simulink model "power_FCV_powertrain_modified"  (R2021b)
settings: Solver=ode23tb  StartTime=0.0  StopTime=1175  RelTol=1e-3  EnableMultiTasking=on
PreLoadFcn:
  | Ts=60e-6;
InitFcn:
  | Pbatt = 25e3;
  | Vbatt = 288;
values from neighbouring files (symbols this model uses):
  Cr = 0.013    [datavehicule.m]    (also in workspace.mat)
  Cx = 0.25    [datavehicule.m]    (also in workspace.mat = 0.65)
  efficency_FC = 0.53    [init.m]    (also in main.m; workspace.mat)
  epsilon = 10^-6    (= 1e-06)    [init.m]    (also in workspace.mat)
  g = 9.81    [datavehicule.m]    (also in init.m; workspace.mat)
  gr = 17/64    (= 0.265625)    [datavehicule.m]    (also in workspace.mat)
  M = 1400    [datavehicule.m]    (also in workspace.mat = 2000)
  p = 0    [datavehicule.m]    (also in workspace.mat)
  Pbatt_2 = 25000    [workspace.mat]
  ro = 1.23    [datavehicule.m]    (also in workspace.mat)
  Sf = 1.6+0.00056*(M-765)    [ForceTrac.m]    (also in workspace.mat = 3.93)
  V = [t, velocity]    [init.m]
undefined symbols (not defined in the file or in its folder): DiscIntNeverNeededParam, Ion, Lithium
libraries: simulink x9, sdl_lib x8, spsCurrentMeasurementLib x6, fl_lib x6, nesl_utility x6, spsSeriesRLCBranchLib x4, AC6DriveInternalModels x3, simulink_extras x2, spsBatteryLib x1, DC6DriveInternalModels x1, spsDiodeLib x1, spsFuelCellStackLib x1
(part 2 of 2)

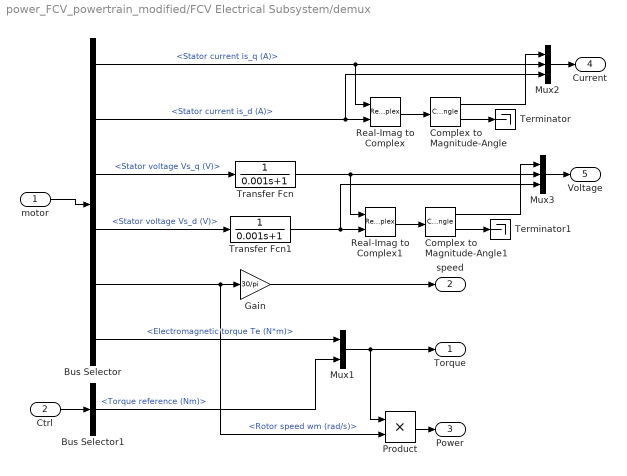
== system power_FCV_powertrain_modified/FCV Electrical Subsystem/demux ==
  motor : Inport
  Ctrl : Inport  Port=2
  Bus Selector : BusSelector  OutputSignals=Stator current is_q (A),Stator current is_d (A),Stator voltage Vs_q (V),Stator voltage Vs_d (V),Rotor speed wm (rad/s),Electromagnetic torque Te (N*m)
  Bus Selector1 : BusSelector  OutputSignals=Torque reference (Nm)
  Complex to Magnitude-Angle : ComplexToMagnitudeAngle
  Complex to Magnitude-Angle1 : ComplexToMagnitudeAngle
  Gain : Gain  Gain=30/pi  SaturateOnIntegerOverflow=on  OutDataTypeStr=Inherit: Same as input  ParamDataTypeStr=Inherit: Same as input
  Mux1 : Mux  Inputs=2
  Mux2 : Mux  Inputs=3
  Mux3 : Mux  Inputs=3
  Product : Product  RndMeth=Zero
  Real-Imag to Complex : RealImagToComplex
  Real-Imag to Complex1 : RealImagToComplex
  Terminator : Terminator
  Terminator1 : Terminator
  Transfer Fcn : TransferFcn  Denominator=[0.001 1]
  Transfer Fcn1 : TransferFcn  Denominator=[0.001 1]
  Torque : Outport
  speed : Outport  Port=2
  Power : Outport  Port=3
  Current : Outport  Port=4
  Voltage : Outport  Port=5
  wires:
  Bus Selector/5 -> Gain/1, Product/2  "<Rotor speed wm (rad/s)>"
  Ctrl/1 -> Bus Selector1/1
  Gain/1 -> speed/1
  Mux1/1 -> Torque/1, Product/1
  motor/1 -> Bus Selector/1
  Mux2/1 -> Current/1
  Product/1 -> Power/1
  Bus Selector/2 -> Real-Imag to Complex/2, Mux2/3  "<Stator current is_d (A)>"
  Bus Selector/1 -> Real-Imag to Complex/1, Mux2/2  "<Stator current is_q (A)>"
  Real-Imag to Complex/1 -> Complex to Magnitude-Angle/1
  Complex to Magnitude-Angle/2 -> Terminator/1
  Complex to Magnitude-Angle/1 -> Mux2/1
  Mux3/1 -> Voltage/1
  Bus Selector/4 -> Transfer Fcn1/1  "<Stator voltage Vs_d (V)>"
  Bus Selector/3 -> Transfer Fcn/1  "<Stator voltage Vs_q (V)>"
  Real-Imag to Complex1/1 -> Complex to Magnitude-Angle1/1
  Complex to Magnitude-Angle1/2 -> Terminator1/1
  Complex to Magnitude-Angle1/1 -> Mux3/1
  Transfer Fcn/1 -> Mux3/2, Real-Imag to Complex1/1
  Transfer Fcn1/1 -> Mux3/3, Real-Imag to Complex1/2
  Bus Selector/6 -> Mux1/1  "<Electromagnetic torque Te (N*m)>"
  Bus Selector1/1 -> Mux1/2  "<Torque reference (Nm)>"

== system power_FCV_powertrain_modified/Energy Management Subsystem/Power Management System/Battery Available Power ==
  P FC : Inport
  P* FC : Inport  Port=2
  Battery recharge : Inport  Port=3
  Power limit : Inport  Port=4
  Add2 : Sum  Inputs=-+
  Compare To Zero : simulink/Logic and Bit Operations/Compare To Zero  relop=~=  OutDataTypeStr=boolean
  Gain : Gain  Gain=-1
  Rate Limiter : RateLimiter  RisingSlewLimit=Pbatt  FallingSlewLimit=-Pbatt  SampleTimeMode=inherited
  Saturation Dynamic : simulink/Discontinuities/Saturation Dynamic  OutMin=[]  OutMax=[]  OutDataTypeStr=Inherit: Same as second input  OutDataType=sfix(16)  OutScaling=2^-10  DoSatur=off
  Switch1 : Switch  Criteria=u2 ~= 0
  Switch2 : Switch  Criteria=u2 ~= 0
  Battery power : Outport
  wires:
  Battery recharge/1 -> Switch1/1, Compare To Zero/1
  Compare To Zero/1 -> Switch1/2, Switch2/2
  P FC/1 -> Add2/1
  Saturation Dynamic/1 -> Battery power/1
  P* FC/1 -> Add2/2
  Add2/1 -> Switch1/3, Switch2/3  "P batt"
  Power limit/1 -> Gain/1, Saturation Dynamic/1
  Gain/1 -> Saturation Dynamic/3
  Switch1/1 -> Rate Limiter/1
  Rate Limiter/1 -> Switch2/1
  Switch2/1 -> Saturation Dynamic/2

== system power_FCV_powertrain_modified/Energy Management Subsystem/Subsystem/iqref1 ==
  In_1 : Inport
  Integral : TransferFcn  Numerator=[I]  Denominator=[1 0]
  Proportional : Gain  Gain=P  SaturateOnIntegerOverflow=on  OutDataTypeStr=Inherit: Same as input  ParamDataTypeStr=Inherit: Same as input
  Saturation : Saturate  UpperLimit=max  LowerLimit=min
  Sum : Sum  InputSameDT=on  SaturateOnIntegerOverflow=on  OutDataTypeStr=Inherit: Same as first input
  Out_1 : Outport  InitialOutput=0  VectorParamsAs1DForOutWhenUnconnected=off
  wires:
  Saturation/1 -> Out_1/1
  Sum/1 -> Saturation/1
  Proportional/1 -> Sum/1
  In_1/1 -> Proportional/1, Integral/1
  Integral/1 -> Sum/2

== system power_FCV_powertrain_modified/Energy Management Subsystem/power_estimation/Rendement ==
  velocity : Inport
  Ft (N) : Inport  Port=2
  MATLAB Function : MATLAB Function  TreatAsAtomicUnit=on
  MATLAB Function1 : MATLAB Function  TreatAsAtomicUnit=on
  MATLAB Function3 : MATLAB Function  TreatAsAtomicUnit=on
  Product : Product
  Power : Outport
  Power_before_transmission : Outport  Port=2
  Power_before_motor : Outport  Port=3
  FC_pw_req : Outport  Port=4
  wires:
  velocity/1 -> Product/1
  Ft (N)/1 -> Product/2
  Product/1 -> MATLAB Function/1(power), MATLAB Function1/1(power), Power/1
  MATLAB Function/1(power_transmission) -> Power_before_transmission/1
  MATLAB Function1/1(power_motor) -> MATLAB Function3/1(power), Power_before_motor/1
  MATLAB Function3/1(power_fuel_cell) -> FC_pw_req/1

== system power_FCV_powertrain_modified/Energy Management Subsystem/power_estimation1/Rendement ==
  velocity : Inport
  Ft (N) : Inport  Port=2
  MATLAB Function : MATLAB Function  TreatAsAtomicUnit=on
  MATLAB Function1 : MATLAB Function  TreatAsAtomicUnit=on
  MATLAB Function3 : MATLAB Function  TreatAsAtomicUnit=on
  Product : Product
  Power : Outport
  Power_before_transmission : Outport  Port=2
  Power_before_motor : Outport  Port=3
  FC_pw_req : Outport  Port=4
  wires:
  velocity/1 -> Product/1
  Ft (N)/1 -> Product/2
  Product/1 -> MATLAB Function/1(power), MATLAB Function1/1(power), Power/1
  MATLAB Function/1(power_transmission) -> Power_before_transmission/1
  MATLAB Function1/1(power_motor) -> MATLAB Function3/1(power), Power_before_motor/1
  MATLAB Function3/1(power_fuel_cell) -> FC_pw_req/1

== system power_FCV_powertrain_modified/FCV Electrical Subsystem/DC-DC converter/Bus DC controller ==
  iref : Inport
  ifc : Inport  Port=2
  Current controller DISCRETE1 : Subsystem  mask(PI controller){Kp=0.0005, Ki=0.1, Ts=Ts}
      mask prompts: Kp "Proportional gain (Kp)"; Ki "Integral gain (Ki)"; Ts "Sample time (s) :"
      mask help: Proportional-Integral Speed Controller
      mask Display: plot(0,0,100,100,[35,35,65],[70,30,30],[35,65],[45,60])
  Duty Cycles : Subsystem
  Fuel cell current limit : TransferFcn  Denominator=[1.5/3 1]
  Mux : Mux  Inputs=2
  Transfer Fcn (with initial outputs)2 : simulink_extras/Additional Linear/Transfer Fcn (with initial outputs)  N=[1]  D="[.0001  1]"  Y0=0  U0=0
  Zero-Order Hold1 : ZeroOrderHold  SampleTime=Ts
  Duty cycle : Outport  InitialOutput=0
  tag scope: I_DCDC=global
  wires:
  Transfer Fcn (with initial outputs)2/1 -> Current controller DISCRETE1/1(ifc), Mux/2
  Duty Cycles/1(dc) -> Duty cycle/1
  Current controller DISCRETE1/1(Ec) -> Duty Cycles/1(Ec)
  Zero-Order Hold1/1 -> Transfer Fcn (with initial outputs)2/1
  iref/1 -> Fuel cell current limit/1
  ifc/1 -> Zero-Order Hold1/1
  Fuel cell current limit/1 -> Current controller DISCRETE1/2(iref), Mux/1
  Mux/1 -> [I_DCDC]

== system power_FCV_powertrain_modified/FCV Electrical Subsystem/DC-DC converter/DC//DC converter ==
  Duty Cycle : Inport
  CBus : spsSeriesRLCBranchLib/Series RLC Branch  LConnTagsString=__new0  RConnTagsString=__new0  BranchType=RC  Resistance=0.2  Inductance=1e-3  SetiL0=off  InitialCurrent=0  Capacitance=1000e-6  Setx0=on  InitialVoltage=200  Measurements=None
  C_FC2 : spsSeriesRLCBranchLib/Series RLC Branch  LConnTagsString=__new0  RConnTagsString=__new0  BranchType=RC  Resistance=0.2  Inductance=1e-3  SetiL0=off  InitialCurrent=0  Capacitance=1000e-6  Setx0=on  InitialVoltage=420  Measurements=None
  Chopper : DC6DriveInternalModels/Chopper (average model)  SnubberResistance=10e3  SnubberCapacitance=inf  Ron=1e-3  ForwardVoltages=[1.3,1.3]  IGBTParameters=[0,0]  converterType=Inverter
      settings: SourceProductBaseCode=PS
  Diode : spsDiodeLib/Diode  Ron=0.001  Lon=0  Vf=0  IC=0  UseSnubber=off  Rs=1e4  Cs=inf  Measurements=off
  L : spsSeriesRLCBranchLib/Series RLC Branch  LConnTagsString=__new0  RConnTagsString=__new0  BranchType=L  Resistance=0.3  Inductance=500e-6  SetiL0=off  InitialCurrent=0  Capacitance=100e-6  Setx0=off  InitialVoltage=0  Measurements=None
  L2 : spsSeriesRLCBranchLib/Series RLC Branch  LConnTagsString=__new0  RConnTagsString=__new0  BranchType=L  Resistance=1  Inductance=1000e-6  SetiL0=on  InitialCurrent=0  Capacitance=100e-6  Setx0=off  InitialVoltage=0  Measurements=None
  i1 : spsCurrentMeasurementLib/Current Measurement  PhasorSimulation=off  OutputType=Complex  PSBequivalent=0
  +Vfc : PMIOPort  Tag=PMCPort  Side=Left
  -Vfc : PMIOPort  Tag=PMCPort  Port=2  Side=Left
  + Vdc : PMIOPort  Tag=PMCPort  Port=3  Side=Right
  - Vdc : PMIOPort  Tag=PMCPort  Port=4  Side=Right
  ifc : Outport
  wires:
  Duty Cycle/1 -> Chopper/1
  i1/1 -> ifc/1  "FC current"
  connections:
  L2/LConn1 -- +Vfc/RConn1
  Chopper/RConn1 -- L/RConn1
  -Vfc/RConn1 -- CBus/RConn1 -- - Vdc/RConn1 -- Chopper/LConn2 -- C_FC2/RConn1
  CBus/LConn1 -- L/LConn1 -- Diode/LConn1
  i1/LConn1 -- L2/RConn1
  Diode/RConn1 -- + Vdc/RConn1
  Chopper/LConn1 -- i1/RConn1 -- C_FC2/LConn1

== system power_FCV_powertrain_modified/FCV Electrical Subsystem/FC Stack /Flow rate regulator Air ==
  Iref : Inport
  Compressor response : TransferFcn  Denominator=[1/3 1]
  Fcn1 : Fcn  Expr=60000*8.3145*(273+95)*400*u(1)/(4*96485*(3*101325)*0.5057*.21)
  Saturation : Saturate  UpperLimit=inf  LowerLimit=60
  flow rate : Outport
  wires:
  Iref/1 -> Fcn1/1
  Saturation/1 -> flow rate/1
  Fcn1/1 -> Compressor response/1
  Compressor response/1 -> Saturation/1

== system power_FCV_powertrain_modified/FCV Electrical Subsystem/FC Stack /Flow rate regulator H2 ==
  Iref : Inport
  Fcn1 : Fcn  Expr=60000*8.3145*(273+95)*400*u(1)/(2*96485*(3*101325)*0.919*.9995)
  Saturation : Saturate  UpperLimit=inf  LowerLimit=1
  flow rate : Outport
  wires:
  Fcn1/1 -> Saturation/1
  Saturation/1 -> flow rate/1
  Iref/1 -> Fcn1/1

== system power_FCV_powertrain_modified/FCV Electrical Subsystem/PM Synchronous Motor Drive This block is based on the AC6 drive block/Measures ==
  Current Measurement : spsCurrentMeasurementLib/Current Measurement  Tag=PoWeRsYsTeMmEaSuReMeNt  PhasorSimulation=off  OutputType=Magnitude  PSBequivalent=0
      settings: AttributesFormatString=\n
  Current Measurement1 : spsCurrentMeasurementLib/Current Measurement  Tag=PoWeRsYsTeMmEaSuReMeNt  PhasorSimulation=off  OutputType=Magnitude  PSBequivalent=0
      settings: AttributesFormatString=\n
  Current Measurement2 : spsCurrentMeasurementLib/Current Measurement  Tag=PoWeRsYsTeMmEaSuReMeNt  PhasorSimulation=off  OutputType=Magnitude  PSBequivalent=0
      settings: AttributesFormatString=\n
  Mux1 : Mux  Inputs=3
  Ta : PMIOPort  Side=Left
  Tb : PMIOPort  Port=2  Side=Left
  Tc : PMIOPort  Port=3  Side=Left
  Mta : PMIOPort  Port=4  Side=Right
  Mtb : PMIOPort  Port=5  Side=Right
  Mtc : PMIOPort  Port=6  Side=Right
  I_abc : Outport
  wires:
  Mux1/1 -> I_abc/1
  Current Measurement2/1 -> Mux1/3
  Current Measurement/1 -> Mux1/1
  Current Measurement1/1 -> Mux1/2
  connections:
  Current Measurement2/RConn1 -- Mtc/RConn1
  Tc/RConn1 -- Current Measurement2/LConn1
  Ta/RConn1 -- Current Measurement/LConn1
  Current Measurement/RConn1 -- Mta/RConn1
  Tb/RConn1 -- Current Measurement1/LConn1
  Current Measurement1/RConn1 -- Mtb/RConn1

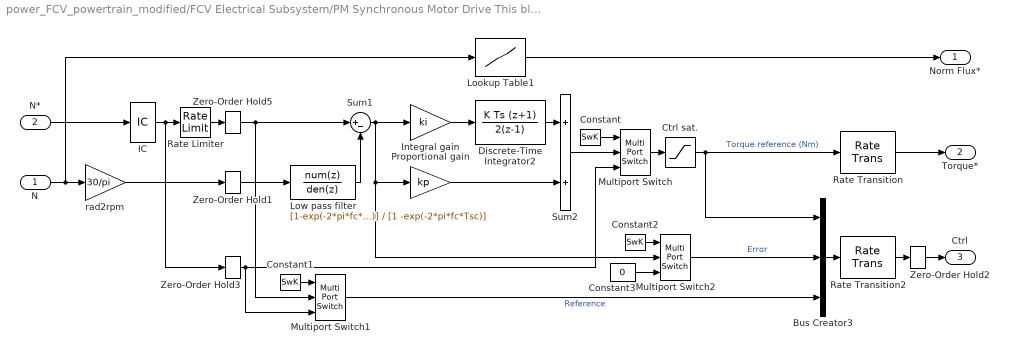
== system power_FCV_powertrain_modified/FCV Electrical Subsystem/PM Synchronous Motor Drive This block is based on the AC6 drive block/Speed Controller ==
  N : Inport
  N* : Inport  Port=2
  Bus Creator3 : BusCreator  Inputs=3
  Constant : Constant  Value=SwK
  Constant1 : Constant  Value=SwK
  Constant2 : Constant  Value=SwK
  Constant3 : Constant  Value=0
  Ctrl sat. : Saturate  UpperLimit=ctrl_sat(2)  LowerLimit=ctrl_sat(1)
  Discrete-Time Integrator2 : DiscreteIntegrator  IntegratorMethod=Integration: Trapezoidal  SampleTime=Tsc  LimitOutput=on  UpperSaturationLimit=ctrl_sat(2)  LowerSaturationLimit=ctrl_sat(1)  ICPrevOutput=DiscIntNeverNeededParam  ICPrevScaledInput=DiscIntNeverNeededParam
  IC : InitialCondition  Value=0
  Integral gain : Gain  Gain=ki  SaturateOnIntegerOverflow=on  OutDataTypeStr=Inherit: Same as input  ParamDataTypeStr=Inherit: Same as input
  Lookup Table1 : Lookup  InputValues=[0 38 40 45 50 60 80 100 120 140 160]*(12500/160/30*pi)  Table="[1 1 0.92 0.86 .83  0.78 0.71 0.675 0.652 0.637 0.612]"
  Low pass filter : DiscreteTransferFcn  Numerator=[1-exp(-2*pi*fc*Tsc)]  Denominator=[1 -exp(-2*pi*fc*Tsc)]  SampleTime=Tsc
  Multiport Switch : MultiPortSwitch  Inputs=2  SaturateOnIntegerOverflow=on
  Multiport Switch1 : MultiPortSwitch  Inputs=2  SaturateOnIntegerOverflow=on
  Multiport Switch2 : MultiPortSwitch  Inputs=2  SaturateOnIntegerOverflow=on
  Proportional gain : Gain  Gain=kp  SaturateOnIntegerOverflow=on  OutDataTypeStr=Inherit: Same as input  ParamDataTypeStr=Inherit: Same as input
  Rate Limiter : RateLimiter  RisingSlewLimit=ramp(2)  FallingSlewLimit=ramp(1)  LinearizeAsGain=off
  Rate Transition : RateTransition
  Rate Transition2 : RateTransition
  Sum1 : Sum  Inputs=|+-  InputSameDT=on  SaturateOnIntegerOverflow=on  OutDataTypeStr=Inherit: Same as first input
  Sum2 : Sum  InputSameDT=on  SaturateOnIntegerOverflow=on  OutDataTypeStr=Inherit: Same as first input
  Zero-Order Hold1 : ZeroOrderHold  SampleTime=Tsc
  Zero-Order Hold2 : ZeroOrderHold  SampleTime=Ts
  Zero-Order Hold3 : ZeroOrderHold  SampleTime=Tsc
  Zero-Order Hold5 : ZeroOrderHold  SampleTime=Tsc
  rad2rpm : Gain  Gain=30/pi  SaturateOnIntegerOverflow=on  OutDataTypeStr=Inherit: Same as input  ParamDataTypeStr=Inherit: Same as input
  Norm Flux* : Outport
  Torque* : Outport  Port=2
  Ctrl : Outport  Port=3
  wires:
  Lookup Table1/1 -> Norm Flux*/1
  rad2rpm/1 -> Zero-Order Hold1/1
  N*/1 -> IC/1
  Ctrl sat./1 -> Rate Transition/1, Bus Creator3/1  "Torque reference (Nm)"
  Integral gain/1 -> Discrete-Time Integrator2/1
  Sum1/1 -> Integral gain/1, Proportional gain/1, Multiport Switch2/2
  N/1 -> Lookup Table1/1, rad2rpm/1
  Discrete-Time Integrator2/1 -> Sum2/1
  Proportional gain/1 -> Sum2/2
  Rate Transition/1 -> Torque*/1
  IC/1 -> Rate Limiter/1, Zero-Order Hold3/1
  Zero-Order Hold1/1 -> Low pass filter/1
  Rate Transition2/1 -> Zero-Order Hold2/1
  Bus Creator3/1 -> Rate Transition2/1
  Zero-Order Hold2/1 -> Ctrl/1
  Low pass filter/1 -> Sum1/2
  Rate Limiter/1 -> Zero-Order Hold5/1
  Zero-Order Hold5/1 -> Sum1/1, Multiport Switch1/2
  Multiport Switch/1 -> Ctrl sat./1
  Constant/1 -> Multiport Switch/1
  Sum2/1 -> Multiport Switch/2
  Constant1/1 -> Multiport Switch1/1
  Zero-Order Hold3/1 -> Multiport Switch/3, Multiport Switch1/3
  Multiport Switch1/1 -> Bus Creator3/3  "Reference"
  Multiport Switch2/1 -> Bus Creator3/2  "Error"
  Constant2/1 -> Multiport Switch2/1
  Constant3/1 -> Multiport Switch2/3

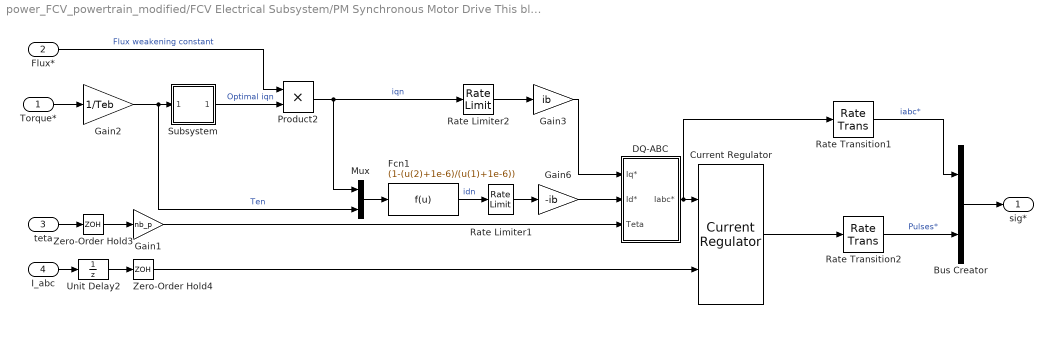
== system power_FCV_powertrain_modified/FCV Electrical Subsystem/PM Synchronous Motor Drive This block is based on the AC6 drive block/VECT ==
  Torque* : Inport
  Flux* : Inport  Port=2
  teta : Inport  Port=3
  I_abc : Inport  Port=4
  Bus Creator : BusCreator  Inputs=2
  Current Regulator : AC6DriveInternalModels/VECT (average model)/Current Regulator  SystemSampleTime=-1  VariantActivationTime=update diagram  Latency=0  AutoFrameSizeCalculation=off
      settings: SourceProductBaseCode=PS
  DQ-ABC : Subsystem
  Fcn1 : Fcn  Expr=(1-(u(2)+1e-6)/(u(1)+1e-6))
  Gain1 : Gain  Gain=nb_p  SaturateOnIntegerOverflow=on  OutDataTypeStr=Inherit: Same as input  ParamDataTypeStr=Inherit: Same as input
  Gain2 : Gain  Gain=1/Teb  SaturateOnIntegerOverflow=on  OutDataTypeStr=Inherit: Same as input  ParamDataTypeStr=Inherit: Same as input
  Gain3 : Gain  Gain=ib  SaturateOnIntegerOverflow=on  OutDataTypeStr=Inherit: Same as input  ParamDataTypeStr=Inherit: Same as input
  Gain6 : Gain  Gain=-ib  SaturateOnIntegerOverflow=on  OutDataTypeStr=Inherit: Same as input  ParamDataTypeStr=Inherit: Same as input
  Mux : Mux  Inputs=2
  Product2 : Product  RndMeth=Zero
  Rate Limiter1 : RateLimiter  RisingSlewLimit=500  FallingSlewLimit=-500  SampleTimeMode=inherited
  Rate Limiter2 : RateLimiter  RisingSlewLimit=500  FallingSlewLimit=-500  SampleTimeMode=inherited
  Rate Transition1 : RateTransition
  Rate Transition2 : RateTransition
  Subsystem : Subsystem
  Unit Delay2 : UnitDelay  SampleTime=-1  HasFrameUpgradeWarning=on
  Zero-Order Hold3 : ZeroOrderHold  SampleTime=Ts_vect
  Zero-Order Hold4 : ZeroOrderHold  SampleTime=Ts_vect
  sig* : Outport
  wires:
  Rate Limiter1/1 -> Gain6/1
  Rate Limiter2/1 -> Gain3/1
  Gain3/1 -> DQ-ABC/1("Iq* ")
  Rate Transition1/1 -> Bus Creator/1  "iabc*"
  Rate Transition2/1 -> Bus Creator/2  "Pulses*"
  Bus Creator/1 -> sig*/1
  Subsystem/1(iqn) -> Product2/2  "Optimal iqn"
  Product2/1 -> Rate Limiter2/1, Mux/1  "iqn"
  Fcn1/1 -> Rate Limiter1/1  "idn"
  Gain6/1 -> DQ-ABC/2("Id* ")
  Flux*/1 -> Product2/1  "Flux weakening constant"
  Mux/1 -> Fcn1/1
  Gain2/1 -> Mux/2, Subsystem/1(Ten)  "Ten"
  Torque*/1 -> Gain2/1
  I_abc/1 -> Unit Delay2/1
  DQ-ABC/1(Iabc*) -> Current Regulator/1, Rate Transition1/1
  Gain1/1 -> DQ-ABC/3(Teta)
  Zero-Order Hold3/1 -> Gain1/1
  teta/1 -> Zero-Order Hold3/1
  Current Regulator/1 -> Rate Transition2/1
  Zero-Order Hold4/1 -> Current Regulator/2
  Unit Delay2/1 -> Zero-Order Hold4/1

== system power_FCV_powertrain_modified/FCV Electrical Subsystem/DC-DC converter/Bus DC controller/Current controller DISCRETE1 ==
  ifc : Inport
  iref : Inport  Port=2
  Ctrl sat. : Saturate  UpperLimit=0.95  LowerLimit=-0.95
  Discrete-Time Integrator : DiscreteIntegrator  IntegratorMethod=Integration: Trapezoidal  SampleTime=Ts  LimitOutput=on  UpperSaturationLimit=1  LowerSaturationLimit=-1  ICPrevOutput=DiscIntNeverNeededParam  ICPrevScaledInput=DiscIntNeverNeededParam
  Integral gain : Gain  Gain=Ki  SaturateOnIntegerOverflow=on  OutDataTypeStr=Inherit: Same as input  ParamDataTypeStr=Inherit: Same as input
  Proportional gain : Gain  Gain=Kp  SaturateOnIntegerOverflow=on  OutDataTypeStr=Inherit: Same as input  ParamDataTypeStr=Inherit: Same as input
  Sum1 : Sum  Inputs=+-  InputSameDT=on  SaturateOnIntegerOverflow=on  OutDataTypeStr=Inherit: Same as first input
  Sum2 : Sum  InputSameDT=on  SaturateOnIntegerOverflow=on  OutDataTypeStr=Inherit: Same as first input
  Ec : Outport  InitialOutput=0
  wires:
  Proportional gain/1 -> Sum2/1
  Integral gain/1 -> Discrete-Time Integrator/1
  Sum1/1 -> Integral gain/1, Proportional gain/1
  ifc/1 -> Sum1/1
  iref/1 -> Sum1/2
  Discrete-Time Integrator/1 -> Sum2/2
  Sum2/1 -> Ctrl sat./1
  Ctrl sat./1 -> Ec/1

== system power_FCV_powertrain_modified/FCV Electrical Subsystem/DC-DC converter/Bus DC controller/Duty Cycles ==
  Ec : Inport
  Add : Sum  Inputs=+-
  Bus Creator2 : BusCreator  Inputs=2
  Constant : Constant
  Duty Cycle : Fcn  Expr=0.5*(u[1]+1)
  dc : Outport
  wires:
  Add/1 -> Bus Creator2/1  "IGBT 2"
  Duty Cycle/1 -> Bus Creator2/2, Add/2  "IGBT I"
  Constant/1 -> Add/1
  Ec/1 -> Duty Cycle/1
  Bus Creator2/1 -> dc/1

== system power_FCV_powertrain_modified/FCV Electrical Subsystem/PM Synchronous Motor Drive This block is based on the AC6 drive block/VECT/DQ-ABC ==
  "Iq* " : Inport
  "Id* " : Inport  Port=2
  Teta : Inport  Port=3
  Fcn : Fcn  Expr=sin(u)
  Fcn1 : Fcn  Expr=cos(u)
  Gain2 : Gain  SaturateOnIntegerOverflow=on  OutDataTypeStr=Inherit: Same as input  ParamDataTypeStr=Inherit: Same as input
  Gain3 : Gain  SaturateOnIntegerOverflow=on  OutDataTypeStr=Inherit: Same as input  ParamDataTypeStr=Inherit: Same as input
  Gain4 : Gain  SaturateOnIntegerOverflow=on  OutDataTypeStr=Inherit: Same as input  ParamDataTypeStr=Inherit: Same as input
  Mux : Mux
  Mux2 : Mux  Inputs=3
  ia : Fcn  Expr=-u[3]*u[2] + u[4]*u[1]
  ib : Fcn  Expr=(-u[1]+1.7320508*u[2])*u[4]*0.5+(u[2]+1.7320508*u[1])*u[3]*0.5
  ic : Sum  Inputs=--  InputSameDT=on  SaturateOnIntegerOverflow=on  OutDataTypeStr=Inherit: Same as first input
  Iabc* : Outport  InitialOutput=0
  wires:
  ib/1 -> ic/1, Gain3/1
  ia/1 -> ic/2, Gain2/1
  Gain2/1 -> Mux2/1
  Gain4/1 -> Mux2/3
  ic/1 -> Gain4/1
  Gain3/1 -> Mux2/2
  "Iq* "/1 -> Mux/4
  "Id* "/1 -> Mux/3
  Teta/1 -> Fcn/1, Fcn1/1
  Mux/1 -> ia/1, ib/1
  Mux2/1 -> Iabc*/1
  Fcn1/1 -> Mux/1
  Fcn/1 -> Mux/2

== system power_FCV_powertrain_modified/FCV Electrical Subsystem/PM Synchronous Motor Drive This block is based on the AC6 drive block/VECT/Subsystem ==
  Ten : Inport
  Abs : Abs
  Fcn2 : Fcn  Expr=(sqrt(4*0.5*u(1)+1)-1)/(2*0.5)
  Product1 : Product  RndMeth=Zero
  Sign : Signum
  iqn : Outport
  wires:
  Product1/1 -> iqn/1
  Ten/1 -> Sign/1, Abs/1
  Sign/1 -> Product1/2
  Fcn2/1 -> Product1/1
  Abs/1 -> Fcn2/1

== matlab function power_FCV_powertrain_modified/Energy Management Subsystem/power_estimation/Rendement/MATLAB Function ==
  data: power input; power_transmission output
function power_transmission = transmission_eff(power)

    power_transmission = power*(1/0.98);
end

== matlab function power_FCV_powertrain_modified/Energy Management Subsystem/power_estimation/MATLAB Function ==
  data: Ft output; velocity input; acceleration input; Facc output; Froul output; Fprof output; Faero output; Force_parameters input
function [ Ft, Facc, Froul , Fprof, Faero ] = ForceTrac( velocity,acceleration,Force_parameters  )
% Calcule les forces necessaires au déplacement d'un vehicule
% time est en sec
% velocity est en m/s
% le vecteur time et velocity ont la même taille et doivent avoir au
% minimum 2 colonnes
Cr = Force_parameters(1);
Cx = Force_parameters(2);
g = Force_parameters(3);
gr = Force_parameters(4);
p = Force_parameters(5);
ro = Force_parameters(6);
M = Force_parameters(7);
Sf = Force_parameters(8);



% Equations mecanique
delta=1.04+0.0025*gr^2;
Facc=delta.*M.*acceleration; % .* multiplication terme à terme
Froul=(M.*g.*Cr);
Fprof=M.*g.*sin(atan(p));
%  Sf=1.6+0.00056*(M-765);
Faero=0.5*ro*Cx*Sf.*velocity.^2;

Ft=Facc+Froul+Fprof+Faero;

% % test
% % 50km/h = 50*1000/3600m/s
% [ Ft Facc Froul Fprof Faero ] = ForceTrac( [0, 10], [50*1000/3600, 50*1000/3600] )
% [ Ft Facc Froul Fprof Faero ] = ForceTrac( [0, 10], [0*1000/3600, 100*1000/3600] )
% [ Ft Facc Froul Fprof Faero ] = ForceTrac( cycle.Time, cycle.Speed.*1000/3600 )

end

== matlab function power_FCV_powertrain_modified/Energy Management Subsystem/power_estimation/Rendement/MATLAB Function1 ==
  data: power input; power_motor output
function power_motor = motor_eff(power)

    power_motor = power*(1/0.89);
end

== matlab function power_FCV_powertrain_modified/Data/H2 Consumption ==
  data: energy_FC input; H2_consumption output
function H2_consumption = fcn(energy_FC)

%calculate the hydrogen consumption in grams, knowing that that the energy density of
%hydrogen is 142MJ/kg which is equal to 142,000J/g
H2_consumption = energy_FC./142000;
H2_consumption = H2_consumption /1000; % to Kg
H2_consumption = H2_consumption*(1000/42); %to L at 700 bar

== matlab function power_FCV_powertrain_modified/Energy Management Subsystem/power_estimation/Rendement/MATLAB Function3 ==
  data: power input; power_fuel_cell output
function power_fuel_cell = fuel_cell_eff(power)

    power_fuel_cell = power*(1/0.53);
end

== matlab function power_FCV_powertrain_modified/Energy Management Subsystem/power_estimation1/MATLAB Function ==
  data: Ft output; velocity input; acceleration input; Facc output; Froul output; Fprof output; Faero output; Force_parameters input
function [ Ft, Facc, Froul , Fprof, Faero ] = ForceTrac( velocity,acceleration,Force_parameters  )
% Calcule les forces necessaires au déplacement d'un vehicule
% time est en sec
% velocity est en m/s
% le vecteur time et velocity ont la même taille et doivent avoir au
% minimum 2 colonnes
Cr = Force_parameters(1);
Cx = Force_parameters(2);
g = Force_parameters(3);
gr = Force_parameters(4);
p = Force_parameters(5);
ro = Force_parameters(6);
M = Force_parameters(7);
Sf = Force_parameters(8);



% Equations mecanique
delta=1.04+0.0025*gr^2;
Facc=delta.*M.*acceleration; % .* multiplication terme à terme
Froul=(M.*g.*Cr);
Fprof=M.*g.*sin(atan(p));
%  Sf=1.6+0.00056*(M-765);
Faero=0.5*ro*Cx*Sf.*velocity.^2;

Ft=Facc+Froul+Fprof+Faero;

% % test
% % 50km/h = 50*1000/3600m/s
% [ Ft Facc Froul Fprof Faero ] = ForceTrac( [0, 10], [50*1000/3600, 50*1000/3600] )
% [ Ft Facc Froul Fprof Faero ] = ForceTrac( [0, 10], [0*1000/3600, 100*1000/3600] )
% [ Ft Facc Froul Fprof Faero ] = ForceTrac( cycle.Time, cycle.Speed.*1000/3600 )

end

== matlab function power_FCV_powertrain_modified/Energy Management Subsystem/power_estimation1/Rendement/MATLAB Function ==
  data: power input; power_transmission output
function power_transmission = transmission_eff(power)

    power_transmission = power*(1/0.98);
end

== matlab function power_FCV_powertrain_modified/Energy Management Subsystem/power_estimation1/Rendement/MATLAB Function1 ==
  data: power input; power_motor output
function power_motor = motor_eff(power)

    power_motor = power*(1/0.89);
end

== matlab function power_FCV_powertrain_modified/Energy Management Subsystem/power_estimation1/Rendement/MATLAB Function3 ==
  data: power input; power_fuel_cell output
function power_fuel_cell = fuel_cell_eff(power)

    power_fuel_cell = power*(1/0.53);
end
